simulink model "invgeo_test"  (Simulink 6.4)
settings: Solver=ode4  StartTime=0.0  StopTime=20  FixedStep=0.01  RelTol=1e-3
libraries: simulink x2
settings Model: LastModifiedBy=Developer

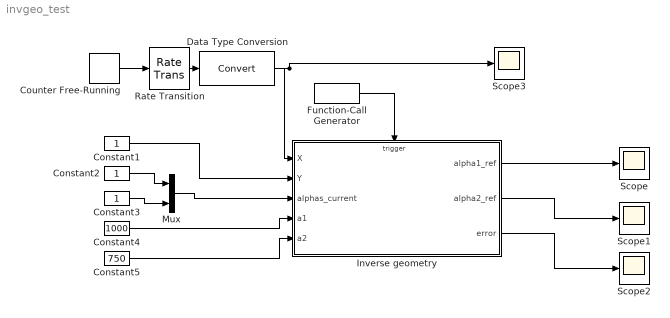
== system invgeo_test ==
  Constant1 : Constant  Value=1  OutDataType=sfix(16)  ConRadixGroup=Use specified scaling  OutScaling=2^0  SampleTime=inf  FramePeriod=inf
  Constant2 : Constant  Value=1  OutDataType=sfix(16)  ConRadixGroup=Use specified scaling  OutScaling=2^0  SampleTime=inf  FramePeriod=inf
  Constant3 : Constant  Value=1  OutDataType=sfix(16)  ConRadixGroup=Use specified scaling  OutScaling=2^0  SampleTime=inf  FramePeriod=inf
  Constant4 : Constant  Value=1000  OutDataType=sfix(16)  ConRadixGroup=Use specified scaling  OutScaling=2^0  SampleTime=inf  FramePeriod=inf
  Constant5 : Constant  Value=750  OutDataType=sfix(16)  ConRadixGroup=Use specified scaling  OutScaling=2^0  SampleTime=inf  FramePeriod=inf
  Counter Free-Running : simulink/Sources/Counter Free-Running  SystemSampleTime=-1  NumBits=16  tsamp=0.01
  Data Type Conversion : DataTypeConversion  OutDataTypeMode=double
  Function-Call Generator : simulink/Ports & Subsystems/Function-Call Generator  sample_time=1  numberOfIterations=100
  Inverse geometry : Subsystem  TreatAsAtomicUnit=on
  Mux : Mux  Inputs=2
  Rate Transition : RateTransition
  Scope{,1..3} (4 alike) : Scope
      Scope2 settings: SaveName=ScopeData2
      Scope3 settings: SaveName=ScopeData3
  wires:
  Counter Free-Running/1 -> Rate Transition/1
  Constant1/1 -> Inverse geometry/2(Y)
  Constant2/1 -> Mux/1
  Constant3/1 -> Mux/2
  Mux/1 -> Inverse geometry/3(alphas_current)
  Constant4/1 -> Inverse geometry/4(a1)
  Constant5/1 -> Inverse geometry/5(a2)
  Inverse geometry/1(alpha1_ref) -> Scope/1
  Inverse geometry/2(alpha2_ref) -> Scope1/1
  Inverse geometry/3(error) -> Scope2/1
  Function-Call Generator/1 -> Inverse geometry/Trigger
  Rate Transition/1 -> Data Type Conversion/1
  Data Type Conversion/1 -> Inverse geometry/1(X), Scope3/1

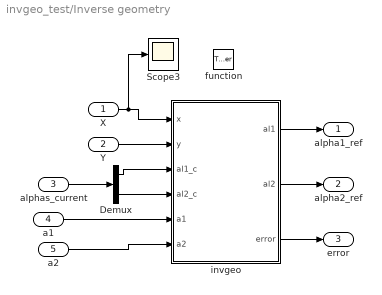
== system invgeo_test/Inverse geometry ==
  X : Inport
  Y : Inport  Port=2
  alphas_current : Inport  Port=3
  a1 : Inport  Port=4
  a2 : Inport  Port=5
  function : TriggerPort  TriggerType=function-call
  Demux : Demux  Outputs=2
  Scope3 : Scope
      settings: SaveName=ScopeData4
  invgeo : Stateflow chart
  alpha1_ref : Outport
  alpha2_ref : Outport  Port=2
  error : Outport  Port=3
  wires:
  X/1 -> invgeo/1(x), Scope3/1
  Y/1 -> invgeo/2(y)
  alphas_current/1 -> Demux/1
  Demux/1 -> invgeo/3(al1_c)
  Demux/2 -> invgeo/4(al2_c)
  a1/1 -> invgeo/5(a1)
  a2/1 -> invgeo/6(a2)
  invgeo/1(al1) -> alpha1_ref/1
  invgeo/2(al2) -> alpha2_ref/1
  invgeo/3(error) -> error/1

== matlab function Inverse geometry/invgeo ==
  data: x input inherited; y input inherited; al1_c input inherited; al2_c input inherited; a1 input inherited; a2 input inherited; al1 output inherited; al2 output inherited; error output inherited
function [al1, al2, error] = invgeo(x, y, al1_c, al2_c, a1, a2)
    
    d = sqrt(x^2 + y^2);
    if ((d^2 > (a1^2 + a2^2)) | (d < (a1 - a2)))
        al1 = al1_c;
        al2 = al2_c;
        error = uint8(1);
        return;
    end
    
    cos_al2 = (x^2 + y^2 - a1^2 - a2^2) / (2 * a1 * a2);
    D = a1 + a2 * cos_al2;
    
    sin_al1_p = (D * y + x * sqrt(x^2 + y^2 - D^2)) / (x^2 + y^2);
    sin_al1_n = (D * y - x * sqrt(x^2 + y^2 - D^2)) / (x^2 + y^2);
    
    cos_al1_p = (D * x + y * sqrt(x^2 + y^2 - D^2)) / (x^2 + y^2);
    cos_al1_n = (D * x - y * sqrt(x^2 + y^2 - D^2)) / (x^2 + y^2);
    
    al1_1 = atan2(sin_al1_p, cos_al1_n);
    
    al1_2 = atan2(sin_al1_n, cos_al1_p);
    
    al2_p = acos(cos_al2);
    al2_n = -al2_p; 
    
    if ( x == (a1 * cos_al1_n + a2 * cos(al1_1 + al2_p)))
        al2_1 = al2_p;
        al2_2 = al2_n;
    else 
       al2_1 = al2_n;
       al2_2 = al2_p;
    end
    
    if (abs(al1_c - al1_1) < abs(al1_c - al1_2))
        al1 = al1_1;
        al2 = al2_1;
    else
        al1 = al1_2;
        al2 = al2_2;
    end
    
    error = uint8(0);  
end
